simulink library "Spring_LeftRight_AsymmetricAirOilPiston"  (R2025a)
settings: Solver=VariableStepAuto  StartTime=0.0  StopTime=10.0  RelTol=1e-3
libraries: fl_lib x2, Spring_AirOilPiston x2
Description:
  | Component of Simscape Vehicle Templates Library
  | 
  | Copyright 2018-2024 The MathWorks, Inc.
settings Model: Creator=smiller  LastModifiedBy=smiller
settings SolverCC: AlgebraicLoopSolver=TrustRegion
settings DataIOCC: ReturnWorkspaceOutputs=off
settings DebuggingCC: UnconnectedInputMsg=warning  UnconnectedOutputMsg=warning  UnconnectedLineMsg=warning  ArithmeticOperatorsInVariantConditions=warning
settings ModelReferenceCC: EnableRefExpFcnMdlSchedulingChecks=on
settings SFSimCC: CustomCodeUndefinedFunction=UseInterfaceOnly
settings RTWCC: GPUComputeCapability=3.5  DLArmComputeVersion=19.05

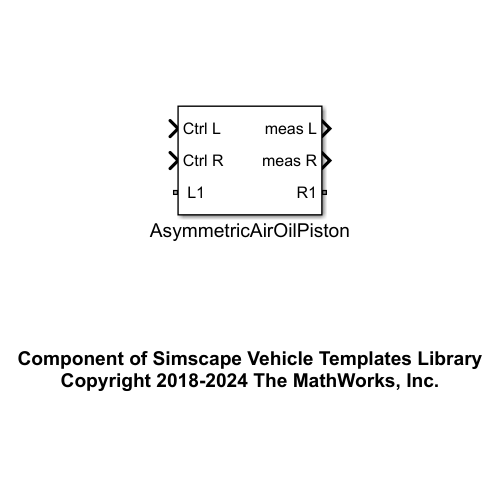
[thumbnail: Simulink's stored preview of the top-level diagram]
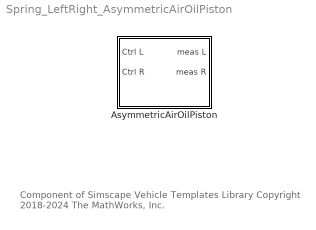
== system Spring_LeftRight_AsymmetricAirOilPiston ==
  note: Component of Simscape Vehicle Templates Library
      | Copyright 2018-2024 The MathWorks, Inc.
  AsymmetricAirOilPiston : Subsystem  VariantControl=Linear  mask(Asymmetric Air Oil Piston Springs){}
      mask help: Air oil piston springs with independent hardpoint parameterization for left and right sides. For spring connections in suspensions that may be asymmetric at design position, such as Panhard rod suspensions.

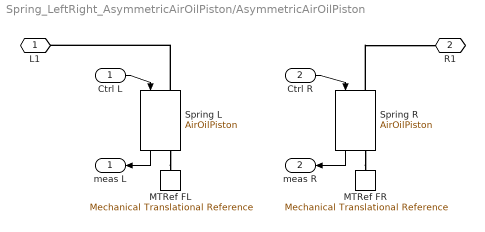
== system Spring_LeftRight_AsymmetricAirOilPiston/AsymmetricAirOilPiston ==
  Ctrl L : Inport
  Ctrl R : Inport  Port=2
  MTRef FL : fl_lib/Mechanical/Translational Elements/Mechanical Translational Reference
  MTRef FR : fl_lib/Mechanical/Translational Elements/Mechanical Translational Reference
  Spring L : Spring_AirOilPiston/AirOilPiston  spr_hp_top=Spring.sTopL.Value  spr_hp_bot=Spring.sBottomL.Value  t_ambient=Spring.Spring.TAmbient.Value  gspr_gas_properties=Spring.Spring.GasProperties  strut_oil_properties=Spring.Strut.OilProperties  gas_chamber_soft_area=Spring.Spring.GasSoft.A.Value  gas_chamber_stiff_area=Spring.Spring.GasStiff.A.Value  gas_chamber_soft_deadvol=Spring.Spring.GasSoft.volDead.Value  gas_chamber_stiff_deadvol=Spring.Spring.GasStiff.volDead.Value  gspr_mass_soft=Spring.Spring.GasSoft.mPiston.Value  gspr_mass_stiff=Spring.Spring.GasStiff.mPiston.Value  gspr_damping_soft=Spring.Spring.GasSoft.b.Value  gspr_damping_stiff=Spring.Spring.GasStiff.b.Value  gas_chamber_soft_x0=Spring.Spring.GasSoft.xInit.Value  gas_chamber_stiff_x0=Spring.Spring.GasStiff.xInit.Value  gas_chamber_soft_p0=Spring.Spring.GasSoft.pInit.Value  gas_chamber_stiff_p0=Spring.Spring.GasStiff.pInit.Value  gspr_cwall_soft=Spring.Spring.GasSoft.CWall.Value  gspr_cwall_stiff=Spring.Spring.GasStiff.CWall.Value  oil_chamber_soft_area=Spring.Spring.OilSoft.A.Value  oil_chamber_stiff_area=Spring.Spring.OilStiff.A.Value  oil_chamber_soft_deadvol=Spring.Spring.OilSoft.volDead.Value  oil_chamber_stiff_deadvol=Spring.Spring.OilStiff.volDead.Value  oil_chamber_soft_x0=Spring.Spring.OilSoft.xInit.Value  oil_chamber_stiff_x0=Spring.Spring.OilStiff.xInit.Value  oil_chamber_soft_p0=Spring.Spring.OilSoft.pInit.Value  oil_chamber_stiff_p0=Spring.Spring.OilStiff.pInit.Value  gsprv_smax_soft=Spring.Spring.ValveSoft.xMaxOpen.Value  gsprv_smax_stiff=Spring.Spring.ValveStiff.xMaxOpen.Value  gsprv_delsmax_soft=Spring.Spring.ValveSoft.xCloseToOpen.Value  gsprv_delsmax_stiff=Spring.Spring.ValveStiff.xCloseToOpen.Value  gsprv_arealeak_soft=Spring.Spring.ValveSoft.areaLeak.Value  gsprv_arealeak_stiff=Spring.Spring.ValveStiff.areaLeak.Value  gsprv_areamax_soft=Spring.Spring.ValveSoft.aMax.Value  gsprv_areamax_stiff=Spring.Spring.ValveStiff.aMax.Value  gsprv_cd_soft=Spring.Spring.ValveSoft.Cd.Value  gsprv_cd_stiff=Spring.Spring.ValveStiff.Cd.Value  gsprv_smooth_soft=Spring.Spring.ValveSoft.smoothFactor.Value  gsprv_smooth_stiff=Spring.Spring.ValveStiff.smoothFactor.Value  gsprva_stroke_soft=Spring.Spring.ValveActuatorSoft.xStroke.Value  gsprva_stroke_stiff=Spring.Spring.ValveActuatorStiff.xStroke.Value  gsprva_ton_soft=Spring.Spring.ValveActuatorSoft.tOn.Value  gsprva_ton_stiff=Spring.Spring.ValveActuatorStiff.tOn.Value  gsprva_toff_soft=Spring.Spring.ValveActuatorSoft.tOff.Value  gsprva_toff_stiff=Spring.Spring.ValveActuatorStiff.tOff.Value  strut_deadvol=Spring.Strut.volDead.Value  strut_area=Spring.Strut.A.Value  strut_x0=Spring.Strut.xInit.Value  strut_frc_colfrc=Spring.Strut.Friction.fCoulomb.Value  strut_frc_brkfrc=Spring.Strut.Friction.fBreakaway.Value  strut_frc_brkvel=Spring.Strut.Friction.vBreakaway.Value  strut_frc_visccoeff=Spring.Strut.Friction.mu.Value  bs_lim_upper=Spring.Endstop.xMax.Value  bs_lim_lower=Spring.Endstop.xMin.Value  bs_k_upper=Spring.Endstop.KxMax.Value  bs_k_lower=Spring.Endstop.KxMin.Value  bs_b_upper=Spring.Endstop.dxMax.Value  bs_b_lower=Spring.Endstop.dxMin.Value  bs_region=Spring.Endstop.xTransition.Value  p_diff_TLU_constant=Spring.Damper.Orifice.pDiff.Value  vol_flow_TLU_constant=Spring.Damper.Orifice.q.Value  dpr_restrarea_comp=Spring.Damper.RestrictionComp.A.Value  dpr_restrarea_reb=Spring.Damper.RestrictionReb.A.Value  dpr_cd_comp=Spring.Damper.RestrictionComp.Cd.Value  dpr_cd_reb=Spring.Damper.RestrictionReb.Cd.Value  dpr_prv_psetdiff_comp=Spring.Damper.PRVComp.pDiff.Value  dpr_prv_psetdiff_reb=Spring.Damper.PRVReb.pDiff.Value  dpr_prv_prange_comp=Spring.Damper.PRVComp.pRange.Value  dpr_prv_prange_reb=Spring.Damper.PRVReb.pRange.Value  dpr_prv_areamax_comp=Spring.Damper.PRVComp.A.Value  dpr_prv_areamax_reb=Spring.Damper.PRVReb.A.Value  dpr_prv_cd_comp=Spring.Damper.PRVComp.Cd.Value  dpr_prv_cd_reb=Spring.Damper.PRVReb.Cd.Value  dpr_cvdvalve_cmpos=Spring.CVDValve.Orifice.x.Value  dpr_cvdvalve_orifice_area=Spring.CVDValve.Orifice.A.Value  dpr_cvdvalve_orifice_pdiff=Spring.CVDValve.Orifice.pDiff.Value  dpr_cvdvalve_pcv_areamax=Spring.CVDValve.PCValve.AMax.Value  dpr_cvdvalve_pcv_prange=Spring.CVDValve.PCValve.pRange.Value  dpr_cvdvalve_arealeak=Spring.CVDValve.PCValve.ALeak.Value  dpr_cvdvalve_cd=Spring.CVDValve.PCValve.Cd.Value  dpr_cvdvalve_act_ts=Spring.CVDValve.tFilt.Value  rh_srcpressure=Spring.RideHeight.pSource.Value  rh_fcv_cmpos_inlet=Spring.RideHeight.OrificeInlet.x.Value  rh_fcv_cmpos_outlet=Spring.RideHeight.OrificeOutlet.x.Value  rh_fcv_orificearea_inlet=Spring.RideHeight.OrificeInlet.A.Value  rh_fcv_orificearea_outlet=Spring.RideHeight.OrificeOutlet.A.Value  rh_fcv_orificepdiff_inlet=Spring.RideHeight.OrificeInlet.pDiff.Value  rh_fcv_orificepdiff_outlet=Spring.RideHeight.OrificeOutlet.pDiff.Value  rh_fcv_pcprange_inlet=Spring.RideHeight.PCValveInlet.pRange.Value  rh_fcv_pcprange_outlet=Spring.RideHeight.PCValveOutlet.pRange.Value  rh_fcv_pcamax_inlet=Spring.RideHeight.PCValveInlet.AMax.Value  rh_fcv_pcamax_outlet=Spring.RideHeight.PCValveOutlet.AMax.Value  rh_fcv_arealeak_inlet=Spring.RideHeight.PCValveInlet.ALeak.Value  rh_fcv_arealeak_outlet=Spring.RideHeight.PCValveOutlet.ALeak.Value  rh_fcv_cd_inlet=Spring.RideHeight.PCValveInlet.Cd.Value  rh_fcv_cd_outlet=Spring.RideHeight.PCValveOutlet.Cd.Value  rh_fcv_smooth_inlet=Spring.RideHeight.PCValveInlet.smoothFactor.Value  rh_fcv_smooth_outlet=Spring.RideHeight.PCValveOutlet.smoothFactor.Value  rh_fcv_tfilt_inlet=Spring.RideHeight.PCValveInlet.tFilt.Value  rh_fcv_tfilt_outlet=Spring.RideHeight.PCValveOutlet.tFilt.Value
  Spring R : Spring_AirOilPiston/AirOilPiston  spr_hp_top=Spring.sTopR.Value  spr_hp_bot=Spring.sBottomR.Value  t_ambient=Spring.Spring.TAmbient.Value  gspr_gas_properties=Spring.Spring.GasProperties  strut_oil_properties=Spring.Strut.OilProperties  gas_chamber_soft_area=Spring.Spring.GasSoft.A.Value  gas_chamber_stiff_area=Spring.Spring.GasStiff.A.Value  gas_chamber_soft_deadvol=Spring.Spring.GasSoft.volDead.Value  gas_chamber_stiff_deadvol=Spring.Spring.GasStiff.volDead.Value  gspr_mass_soft=Spring.Spring.GasSoft.mPiston.Value  gspr_mass_stiff=Spring.Spring.GasStiff.mPiston.Value  gspr_damping_soft=Spring.Spring.GasSoft.b.Value  gspr_damping_stiff=Spring.Spring.GasStiff.b.Value  gas_chamber_soft_x0=Spring.Spring.GasSoft.xInit.Value  gas_chamber_stiff_x0=Spring.Spring.GasStiff.xInit.Value  gas_chamber_soft_p0=Spring.Spring.GasSoft.pInit.Value  gas_chamber_stiff_p0=Spring.Spring.GasStiff.pInit.Value  gspr_cwall_soft=Spring.Spring.GasSoft.CWall.Value  gspr_cwall_stiff=Spring.Spring.GasStiff.CWall.Value  oil_chamber_soft_area=Spring.Spring.OilSoft.A.Value  oil_chamber_stiff_area=Spring.Spring.OilStiff.A.Value  oil_chamber_soft_deadvol=Spring.Spring.OilSoft.volDead.Value  oil_chamber_stiff_deadvol=Spring.Spring.OilStiff.volDead.Value  oil_chamber_soft_x0=Spring.Spring.OilSoft.xInit.Value  oil_chamber_stiff_x0=Spring.Spring.OilStiff.xInit.Value  oil_chamber_soft_p0=Spring.Spring.OilSoft.pInit.Value  oil_chamber_stiff_p0=Spring.Spring.OilStiff.pInit.Value  gsprv_smax_soft=Spring.Spring.ValveSoft.xMaxOpen.Value  gsprv_smax_stiff=Spring.Spring.ValveStiff.xMaxOpen.Value  gsprv_delsmax_soft=Spring.Spring.ValveSoft.xCloseToOpen.Value  gsprv_delsmax_stiff=Spring.Spring.ValveStiff.xCloseToOpen.Value  gsprv_arealeak_soft=Spring.Spring.ValveSoft.areaLeak.Value  gsprv_arealeak_stiff=Spring.Spring.ValveStiff.areaLeak.Value  gsprv_areamax_soft=Spring.Spring.ValveSoft.aMax.Value  gsprv_areamax_stiff=Spring.Spring.ValveStiff.aMax.Value  gsprv_cd_soft=Spring.Spring.ValveSoft.Cd.Value  gsprv_cd_stiff=Spring.Spring.ValveStiff.Cd.Value  gsprv_smooth_soft=Spring.Spring.ValveSoft.smoothFactor.Value  gsprv_smooth_stiff=Spring.Spring.ValveStiff.smoothFactor.Value  gsprva_stroke_soft=Spring.Spring.ValveActuatorSoft.xStroke.Value  gsprva_stroke_stiff=Spring.Spring.ValveActuatorStiff.xStroke.Value  gsprva_ton_soft=Spring.Spring.ValveActuatorSoft.tOn.Value  gsprva_ton_stiff=Spring.Spring.ValveActuatorStiff.tOn.Value  gsprva_toff_soft=Spring.Spring.ValveActuatorSoft.tOff.Value  gsprva_toff_stiff=Spring.Spring.ValveActuatorStiff.tOff.Value  strut_deadvol=Spring.Strut.volDead.Value  strut_area=Spring.Strut.A.Value  strut_x0=Spring.Strut.xInit.Value  strut_frc_colfrc=Spring.Strut.Friction.fCoulomb.Value  strut_frc_brkfrc=Spring.Strut.Friction.fBreakaway.Value  strut_frc_brkvel=Spring.Strut.Friction.vBreakaway.Value  strut_frc_visccoeff=Spring.Strut.Friction.mu.Value  bs_lim_upper=Spring.Endstop.xMax.Value  bs_lim_lower=Spring.Endstop.xMin.Value  bs_k_upper=Spring.Endstop.KxMax.Value  bs_k_lower=Spring.Endstop.KxMin.Value  bs_b_upper=Spring.Endstop.dxMax.Value  bs_b_lower=Spring.Endstop.dxMin.Value  bs_region=Spring.Endstop.xTransition.Value  p_diff_TLU_constant=Spring.Damper.Orifice.pDiff.Value  vol_flow_TLU_constant=Spring.Damper.Orifice.q.Value  dpr_restrarea_comp=Spring.Damper.RestrictionComp.A.Value  dpr_restrarea_reb=Spring.Damper.RestrictionReb.A.Value  dpr_cd_comp=Spring.Damper.RestrictionComp.Cd.Value  dpr_cd_reb=Spring.Damper.RestrictionReb.Cd.Value  dpr_prv_psetdiff_comp=Spring.Damper.PRVComp.pDiff.Value  dpr_prv_psetdiff_reb=Spring.Damper.PRVReb.pDiff.Value  dpr_prv_prange_comp=Spring.Damper.PRVComp.pRange.Value  dpr_prv_prange_reb=Spring.Damper.PRVReb.pRange.Value  dpr_prv_areamax_comp=Spring.Damper.PRVComp.A.Value  dpr_prv_areamax_reb=Spring.Damper.PRVReb.A.Value  dpr_prv_cd_comp=Spring.Damper.PRVComp.Cd.Value  dpr_prv_cd_reb=Spring.Damper.PRVReb.Cd.Value  dpr_cvdvalve_cmpos=Spring.CVDValve.Orifice.x.Value  dpr_cvdvalve_orifice_area=Spring.CVDValve.Orifice.A.Value  dpr_cvdvalve_orifice_pdiff=Spring.CVDValve.Orifice.pDiff.Value  dpr_cvdvalve_pcv_areamax=Spring.CVDValve.PCValve.AMax.Value  dpr_cvdvalve_pcv_prange=Spring.CVDValve.PCValve.pRange.Value  dpr_cvdvalve_arealeak=Spring.CVDValve.PCValve.ALeak.Value  dpr_cvdvalve_cd=Spring.CVDValve.PCValve.Cd.Value  dpr_cvdvalve_act_ts=Spring.CVDValve.tFilt.Value  rh_srcpressure=Spring.RideHeight.pSource.Value  rh_fcv_cmpos_inlet=Spring.RideHeight.OrificeInlet.x.Value  rh_fcv_cmpos_outlet=Spring.RideHeight.OrificeOutlet.x.Value  rh_fcv_orificearea_inlet=Spring.RideHeight.OrificeInlet.A.Value  rh_fcv_orificearea_outlet=Spring.RideHeight.OrificeOutlet.A.Value  rh_fcv_orificepdiff_inlet=Spring.RideHeight.OrificeInlet.pDiff.Value  rh_fcv_orificepdiff_outlet=Spring.RideHeight.OrificeOutlet.pDiff.Value  rh_fcv_pcprange_inlet=Spring.RideHeight.PCValveInlet.pRange.Value  rh_fcv_pcprange_outlet=Spring.RideHeight.PCValveOutlet.pRange.Value  rh_fcv_pcamax_inlet=Spring.RideHeight.PCValveInlet.AMax.Value  rh_fcv_pcamax_outlet=Spring.RideHeight.PCValveOutlet.AMax.Value  rh_fcv_arealeak_inlet=Spring.RideHeight.PCValveInlet.ALeak.Value  rh_fcv_arealeak_outlet=Spring.RideHeight.PCValveOutlet.ALeak.Value  rh_fcv_cd_inlet=Spring.RideHeight.PCValveInlet.Cd.Value  rh_fcv_cd_outlet=Spring.RideHeight.PCValveOutlet.Cd.Value  rh_fcv_smooth_inlet=Spring.RideHeight.PCValveInlet.smoothFactor.Value  rh_fcv_smooth_outlet=Spring.RideHeight.PCValveOutlet.smoothFactor.Value  rh_fcv_tfilt_inlet=Spring.RideHeight.PCValveInlet.tFilt.Value  rh_fcv_tfilt_outlet=Spring.RideHeight.PCValveOutlet.tFilt.Value
  " L1" : PMIOPort  Side=Left
  R1 : PMIOPort  Port=2  Side=Right
  meas L : Outport  VectorParamsAs1DForOutWhenUnconnected=off
  meas R : Outport  Port=2  VectorParamsAs1DForOutWhenUnconnected=off
  wires:
  Ctrl L/1 -> Spring L/1
  Spring L/1 -> meas L/1
  Spring R/1 -> meas R/1
  Ctrl R/1 -> Spring R/1
  connections:
  Spring L/RConn1 -- MTRef FL/LConn1
  Spring R/RConn1 -- MTRef FR/LConn1
  Spring L/LConn1 -- " L1"/RConn1
  Spring R/LConn1 -- R1/RConn1
